simulink model "DTC_Load"  (R2020a)
settings: Solver=VariableStepAuto  StartTime=0.0  StopTime=1  RelTol=1e-3
undefined symbols (not defined in the file): sigbuilder_block
libraries: powerlib x7, simulink x4, mcbcontrolslib x3, mcbpositiondecoderlib x2, powerlib_meascontrol x1
settings Model: Creator=rahee  LastModifiedBy=rahee
settings SolverCC: AlgebraicLoopSolver=LineSearch
settings DataIOCC: ReturnWorkspaceOutputs=off

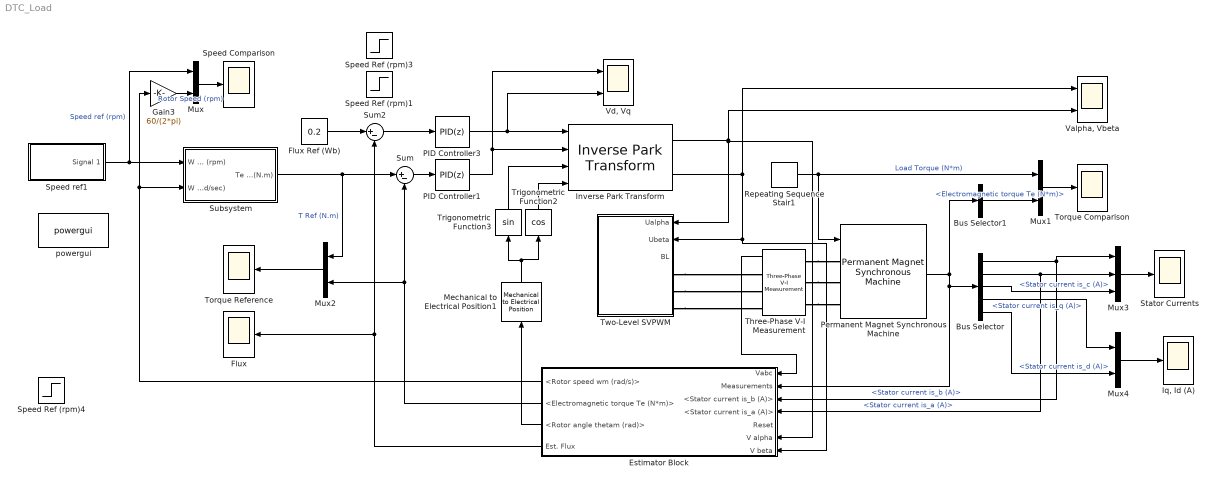
== system DTC_Load ==
  Bus Selector : BusSelector  OutputSignals=Stator current is_b (A),Stator current is_a (A),Stator current is_c (A),Stator current is_q (A),Stator current is_d (A)
  Bus Selector1 : BusSelector  OutputSignals=Electromagnetic torque Te (N*m)
  Estimator Block : Subsystem
  Flux : Scope
  Flux Ref (Wb) : Constant  Value=0.2
  Gain3 : Gain  Gain=60/(2*pi)
  Inverse Park Transform : mcbcontrolslib/Inverse Park Transform  AxisAlignment=D-axis
  "Iq, Id (A)" : Scope
  Mechanical to Electrical Position1 : mcbpositiondecoderlib/Mechanical to Electrical Position  LabelModeActiveChoice=floating-point  NrPP=3  selectedRange=Radians  MechOfstInputType=Specify via dialog  mechOffsetIn=0  maxAngleIn=2*pi  InputDataType=double  VariantSelect=floating-point
      settings: SourceProductBaseCode=MT
  Mux{,1..2,4} (4 alike) : Mux  Inputs=2
  Mux3 : Mux  Inputs=3
  PID Controller1 : simulink/Continuous/PID Controller  Controller=PID  Form=Parallel  TimeDomain=Discrete-time  UseExternalTs=off  SampleTime=-1  IntegratorMethod=Forward Euler  FilterMethod=Forward Euler  ControllerParametersSource=internal  P=8  I=2  D=0  UseFilter=on  N=100  TunerSelectOption=Transfer Function Based (PID Tuner App)  InitialConditionSource=internal  InitialConditionForIntegrator=0  InitialConditionForFilter=0  DifferentiatorICPrevScaledInput=0  ExternalReset=none  TrackingMode=off  Kt=1  LimitOutput=on  UpperSaturationLimit=300  LowerSaturationLimit=-300  LinearizeAsGain=on  AntiWindupMode=clamping  Kb=1  POutMin=[]  POutMax=[]  IOutMin=[]  IOutMax=[]  DOutMin=[]  DOutMax=[]  NOutMin=[]  NOutMax=[]  SumOutMin=[]  SumOutMax=[]  SaturationOutMin=[]  SaturationOutMax=[]  PParamMin=[]  PParamMax=[]  IParamMin=[]  IParamMax=[]  DParamMin=[]  DParamMax=[]  NParamMin=[]  NParamMax=[]  KbParamMin=[]  KbParamMax=[]  KtParamMin=[]  KtParamMax=[]  KbOutMin=[]  KbOutMax=[]  KtOutMin=[]  KtOutMax=[]  IntegratorOutMin=[]  IntegratorOutMax=[]  FilterOutMin=[]  FilterOutMax=[]  SumI1OutMin=[]  SumI1OutMax=[]  SumI2OutMin=[]  SumI2OutMax=[]  SumI3OutMin=[]  SumI3OutMax=[]  SumI4OutMin=[]  SumI4OutMax=[]  SumDOutMin=[]  SumDOutMax=[]  DifferentiatorOutMin=[]  DifferentiatorOutMax=[]  FilterDiffOutCoefMin=[]  FilterDiffOutCoefMax=[]  ReciprocalOutMin=[]  ReciprocalOutMax=[]  SumDenOutMin=[]  SumDenOutMax=[]  SumNumOutMin=[]  SumNumOutMax=[]  DivideOutMin=[]  DivideOutMax=[]  UdiffTsProdOutMin=[]  UdiffTsProdOutMax=[]  NTsProdOutMin=[]  NTsProdOutMax=[]  UintegralTsProdOutMin=[]  UintegralTsProdOutMax=[]  UngainTsProdOutMin=[]  UngainTsProdOutMax=[]  IntegratorContinuousStateAttributes=''  IntegratorStateMustResolveToSignalObject=off  IntegratorRTWStateStorageClass=Auto  FilterContinuousStateAttributes=''  FilterStateMustResolveToSignalObject=off  FilterRTWStateStorageClass=Auto  ParallelPVariant=InternalParameters  IdealPVariant=Disabled  IVariant=InternalParameters  DVariant=InternalParameters  IntegratorVariant=Discrete  SatVariant=Enabled  AWVariant=DiscClampingParallel  PCopyVariant=Disabled  TRVariant=Disabled  FdbkBlocksVariant=Forward  IdealPFdbkVariant=Disabled  SatFdbkVariant=Disabled  DerivativeFilterVariant=ForwardEulerFilter  NVariant=InternalParameters  NCopyVariant=Disabled  FilterICVariant=InternalICsFilter  IntegratorICVariant=InternalICs  ExternalResetVariant=Disabled  TRSumVariant=Passthrough  SumFdbkVariant=Disabled  SumVariant=Sum_PID  TsampFilterVariant=InternalTs  TsampNgainVariant=Passthrough  TsampIntegralVariant=Passthrough
  PID Controller3 : simulink/Continuous/PID Controller  Controller=PID  Form=Parallel  TimeDomain=Discrete-time  UseExternalTs=off  SampleTime=-1  IntegratorMethod=Forward Euler  FilterMethod=Forward Euler  ControllerParametersSource=internal  P=20  I=12  D=0  UseFilter=on  N=100  TunerSelectOption=Transfer Function Based (PID Tuner App)  InitialConditionSource=internal  InitialConditionForIntegrator=0  InitialConditionForFilter=0  DifferentiatorICPrevScaledInput=0  ExternalReset=none  TrackingMode=off  Kt=1  LimitOutput=on  UpperSaturationLimit=300  LowerSaturationLimit=-300  LinearizeAsGain=on  AntiWindupMode=clamping  Kb=1  POutMin=[]  POutMax=[]  IOutMin=[]  IOutMax=[]  DOutMin=[]  DOutMax=[]  NOutMin=[]  NOutMax=[]  SumOutMin=[]  SumOutMax=[]  SaturationOutMin=[]  SaturationOutMax=[]  PParamMin=[]  PParamMax=[]  IParamMin=[]  IParamMax=[]  DParamMin=[]  DParamMax=[]  NParamMin=[]  NParamMax=[]  KbParamMin=[]  KbParamMax=[]  KtParamMin=[]  KtParamMax=[]  KbOutMin=[]  KbOutMax=[]  KtOutMin=[]  KtOutMax=[]  IntegratorOutMin=[]  IntegratorOutMax=[]  FilterOutMin=[]  FilterOutMax=[]  SumI1OutMin=[]  SumI1OutMax=[]  SumI2OutMin=[]  SumI2OutMax=[]  SumI3OutMin=[]  SumI3OutMax=[]  SumI4OutMin=[]  SumI4OutMax=[]  SumDOutMin=[]  SumDOutMax=[]  DifferentiatorOutMin=[]  DifferentiatorOutMax=[]  FilterDiffOutCoefMin=[]  FilterDiffOutCoefMax=[]  ReciprocalOutMin=[]  ReciprocalOutMax=[]  SumDenOutMin=[]  SumDenOutMax=[]  SumNumOutMin=[]  SumNumOutMax=[]  DivideOutMin=[]  DivideOutMax=[]  UdiffTsProdOutMin=[]  UdiffTsProdOutMax=[]  NTsProdOutMin=[]  NTsProdOutMax=[]  UintegralTsProdOutMin=[]  UintegralTsProdOutMax=[]  UngainTsProdOutMin=[]  UngainTsProdOutMax=[]  IntegratorContinuousStateAttributes=''  IntegratorStateMustResolveToSignalObject=off  IntegratorRTWStateStorageClass=Auto  FilterContinuousStateAttributes=''  FilterStateMustResolveToSignalObject=off  FilterRTWStateStorageClass=Auto  ParallelPVariant=InternalParameters  IdealPVariant=Disabled  IVariant=InternalParameters  DVariant=InternalParameters  IntegratorVariant=Discrete  SatVariant=Enabled  AWVariant=DiscClampingParallel  PCopyVariant=Disabled  TRVariant=Disabled  FdbkBlocksVariant=Forward  IdealPFdbkVariant=Disabled  SatFdbkVariant=Disabled  DerivativeFilterVariant=ForwardEulerFilter  NVariant=InternalParameters  NCopyVariant=Disabled  FilterICVariant=InternalICsFilter  IntegratorICVariant=InternalICs  ExternalResetVariant=Disabled  TRSumVariant=Passthrough  SumFdbkVariant=Disabled  SumVariant=Sum_PID  TsampFilterVariant=InternalTs  TsampNgainVariant=Passthrough  TsampIntegralVariant=Passthrough
  Permanent Magnet Synchronous Machine : powerlib/Machines/Permanent Magnet Synchronous Machine  NbPhases=3  FluxDistribution=Sinusoidal  RotorType=Salient-pole  MechanicalLoad=Torque Tm  PresetModel=No  ShowDetailedParameters=on  MeasurementBus=off  Resistance=2  Inductance=8.5e-3  dqInductances=[53.24e-3, 53.24e-3]  La=0.000395  MachineConstant=Torque Constant (N.m / A_peak)  Flux=0.20331  VoltageCst=110.6297  TorqueCst=0.9149  Flat=120  Mechanical=[0.0036 0.0011 3 0]  PolePairs=4  InitialConditions=[0,0, 0,0]  InitialConditions5ph=[0 0 0 0 0 0]  RefAngle=Aligned with phase A axis (original Park)  IterativeDiscreteModel=Trapezoidal non iterative  TsBlock=-1  TsPowergui=0
  Repeating Sequence Stair1 : simulink/Sources/Repeating Sequence Stair  OutValues=[0 0].'  tsamp=0.2  OutMin=[]  OutMax=[]  OutDataTypeStr=double  OutputDataTypeScalingMode=double  OutDataType=fixdt(0,8)  ConRadixGroup=Best Precision: Vector-wise  OutScaling=2^-12
  Speed Comparison : Scope
  Speed Ref (rpm)1 : Step  Time=0.02  After=200  SampleTime=0
  Speed Ref (rpm)3 : Step  Time=0.02  Before=0.2  After=0.2  SampleTime=0
  Speed Ref (rpm)4 : Step  Time=0.1  After=800  SampleTime=0
  Speed ref1 : Subsystem  Tag=STV Subsys  LoadFcn=sigbuilder_block('load',[5.4 30 1141.2 522.6 ]);  StartFcn=sigbuilder_block('start');  StopFcn=sigbuilder_block('stop');  ClipboardFcn=sigbuilder_block('clipboard');  mask(Sigbuilder block){tuvar=[0:10]}
      mask help: Simulink:masks:SigbuilderBlock_MD
      mask init:
      | if ~strcmp(get_param(bdroot(gcbh),'SimulationStatus'),'stopped') tuvar = sigbuilder_block('maskInit'); end
      settings: CopyFcn=sigbuilder_block('copy');  DeleteFcn=sigbuilder_block('delete');  ModelCloseFcn=sigbuilder_block('modelClose');  PreSaveFcn=sigbuilder_block('preSave');  PauseFcn=sigbuilder_block('pause');  ContinueFcn=sigbuilder_block('continue');  NameChangeFcn=sigbuilder_block('namechange');  OpenFcn=sigbuilder_block('open',[5.4 30 1141.2 522.6 ]);  CloseFcn=sigbuilder_block('close');
      mask Display: plot(0, 0, 100, 100,[2, 2, 32, 32, 2], [68, 8, 8, 68, 68],[32, 2], [38, 38], [32, 19, 2],[53, 60, 44], [32, 17, 17, 2],[16, 16, 31, 31]);txt = getActiveGroup(gcbh);text(2, 100, txt,'verticalAlignment', 'top');
  Stator Currents : Scope
  Subsystem : Subsystem
  Sum : Sum  Inputs=|+-
  Sum2 : Sum  Inputs=|+-
  Three-Phase V-I Measurement : powerlib/Measurements/Three-Phase V-I Measurement  VoltageMeasurement=phase-to-ground  SetLabelV=off  LabelV=Vabc  Vpu=off  VpuLL=off  CurrentMeasurement=no  SetLabelI=off  LabelI=Iabc  Ipu=off  Pbase=100e6  Vbase=500e3  OutputType=Complex  PhasorSimulation=off  PSBequivalent=0
  Torque Comparison : Scope
  Torque Reference : Scope
  Trigonometric Function2 : Trigonometry  Operator=cos
  Trigonometric Function3 : Trigonometry
  Two-Level SVPWM : Subsystem
  "Valpha, Vbeta" : Scope  NumInputPorts=2
  "Vd, Vq" : Scope  NumInputPorts=2
  powergui : powerlib/powergui  Priority=1  SimulationMode=Discrete  SampleTime=5e-6  frequency=60  Iterations=50  frequencyindice=0  Pbase=100e6  ErrMax=1e-4  UnitsV=kV  UnitsW=MW  buscounter=0  FunctionMessages=off  echomessages=off  EnableUseOfTLC=off  CurrentSourceSwitches=off  DisableSnubberDevices=off  DisableRonSwitches=off  DisableVfSwitches=off  DisplayEquations=off  AutomaticDiscreteSolvers=off  SolverType=Tustin/Backward Euler (TBE)  Interpol=off  ExternalGateDelay=off  methode=off  Ts=100  x0status=blocks  SPID=on  SwTol=0  HookPort=off  NonlinearTolerance=1e-4  nMaxIteration=100  ContinueOnMaxIteration=off  RestoreLinks=warning  ResistiveCurrentMeasurement=off  Frange=[0:2:500]  Ylog=off  Xlog=on  ShowGrid=off  save=off  variable=ZData  structure=0  ZoomFFT=off  StartTime=0.0  cycles=1  DisplayStyle=1  fundamental=60  FreqAxis=off  MaxFrequency=1000  frequencyindicesteady=1  RmsSteady=1  display=off
  wires:
  Permanent Magnet Synchronous Machine/1 -> Estimator Block/2(Measurements), Bus Selector/1, Bus Selector1/1
  Bus Selector/1 -> Estimator Block/3(<Stator current is_b (A)>), Mux3/1  "<Stator current is_b (A)>"
  Bus Selector/2 -> Mux3/2, Estimator Block/4(<Stator current is_a (A)>)  "<Stator current is_a (A)>"
  Inverse Park Transform/1 -> Estimator Block/6(V alpha), Two-Level SVPWM/1(Ualpha), "Valpha, Vbeta"/2
  Inverse Park Transform/2 -> Estimator Block/7(V beta), Two-Level SVPWM/2(Ubeta), "Valpha, Vbeta"/1
  Sum/1 -> PID Controller1/1
  Sum2/1 -> PID Controller3/1
  Trigonometric Function2/1 -> Inverse Park Transform/4
  Trigonometric Function3/1 -> Inverse Park Transform/3
  Flux Ref (Wb)/1 -> Sum2/1
  PID Controller3/1 -> Inverse Park Transform/1, "Vd, Vq"/2
  PID Controller1/1 -> Inverse Park Transform/2, "Vd, Vq"/1
  Mechanical to Electrical Position1/1 -> Trigonometric Function3/1, Trigonometric Function2/1
  Mux/1 -> Speed Comparison/1
  Mux1/1 -> Torque Comparison/1
  Bus Selector1/1 -> Mux1/2  "<Electromagnetic torque Te (N*m)>"
  Gain3/1 -> Mux/2  "Rotor Speed (rpm)"
  Estimator Block/4(Est. Flux) -> Flux/1, Sum2/2
  Estimator Block/2(<Electromagnetic torque Te (N*m)>) -> Mux2/2, Sum/2
  Estimator Block/1(<Rotor speed wm (rad/s)>) -> Subsystem/2(W meas (rad/sec)), Gain3/1
  Three-Phase V-I Measurement/1 -> Estimator Block/1(Vabc)
  Estimator Block/3(<Rotor angle thetam (rad)>) -> Mechanical to Electrical Position1/1
  Mux2/1 -> Torque Reference/1
  Subsystem/1(Te Ref (N.m)) -> Mux2/1, Sum/1  "T Ref (N.m)"
  Speed ref1/1(Signal 1) -> Mux/1, Subsystem/1(W Ref (rpm))  "Speed ref (rpm)"
  Repeating Sequence Stair1/1 -> Mux1/1, Permanent Magnet Synchronous Machine/1  "Load Torque (N*m)"
  Mux3/1 -> Stator Currents/1
  Bus Selector/3 -> Mux3/3  "<Stator current is_c (A)>"
  Mux4/1 -> "Iq, Id (A)"/1
  Bus Selector/4 -> Mux4/1  "<Stator current is_q (A)>"
  Bus Selector/5 -> Mux4/2  "<Stator current is_d (A)>"
  connections:
  Three-Phase V-I Measurement/LConn1 -- Permanent Magnet Synchronous Machine/LConn1
  Three-Phase V-I Measurement/LConn2 -- Permanent Magnet Synchronous Machine/LConn2
  Three-Phase V-I Measurement/LConn3 -- Permanent Magnet Synchronous Machine/LConn3
  Two-Level SVPWM/LConn1 -- Three-Phase V-I Measurement/RConn1
  Two-Level SVPWM/LConn2 -- Three-Phase V-I Measurement/RConn2
  Two-Level SVPWM/LConn3 -- Three-Phase V-I Measurement/RConn3

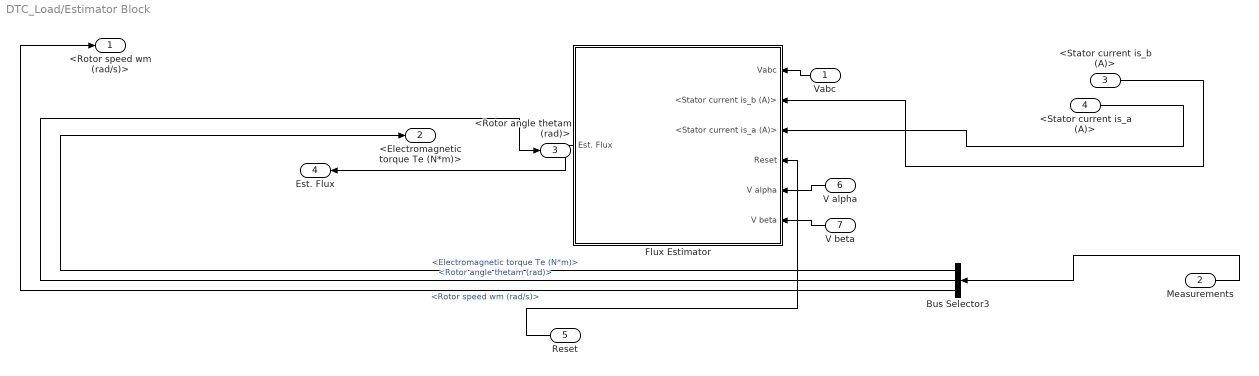
== system DTC_Load/Estimator Block ==
  Vabc : Inport
  Measurements : Inport  Port=2
  <Stator current is_b (A)> : Inport  Port=3
  <Stator current is_a (A)> : Inport  Port=4
  Reset : Inport  Port=5
  V alpha : Inport  Port=6
  V beta : Inport  Port=7
  Bus Selector3 : BusSelector  OutputSignals=Electromagnetic torque Te (N*m),Rotor angle thetam (rad),Rotor speed wm (rad/s)
  Flux Estimator : Subsystem
  <Rotor speed wm (rad/s)> : Outport
  <Electromagnetic torque Te (N*m)> : Outport  Port=2
  <Rotor angle thetam (rad)> : Outport  Port=3
  Est. Flux : Outport  Port=4
  wires:
  Measurements/1 -> Bus Selector3/1
  Bus Selector3/3 -> <Rotor speed wm (rad/s)>/1  "<Rotor speed wm (rad/s)>"
  Flux Estimator/1(Est. Flux) -> Est. Flux/1
  Bus Selector3/1 -> <Electromagnetic torque Te (N*m)>/1  "<Electromagnetic torque Te (N*m)>"
  <Stator current is_a (A)>/1 -> Flux Estimator/3(<Stator current is_a (A)>)
  <Stator current is_b (A)>/1 -> Flux Estimator/2(<Stator current is_b (A)>)
  Vabc/1 -> Flux Estimator/1(Vabc)
  Reset/1 -> Flux Estimator/4(Reset)
  Bus Selector3/2 -> <Rotor angle thetam (rad)>/1  "<Rotor angle thetam (rad)>"
  V alpha/1 -> Flux Estimator/5(V alpha)
  V beta/1 -> Flux Estimator/6(V beta)

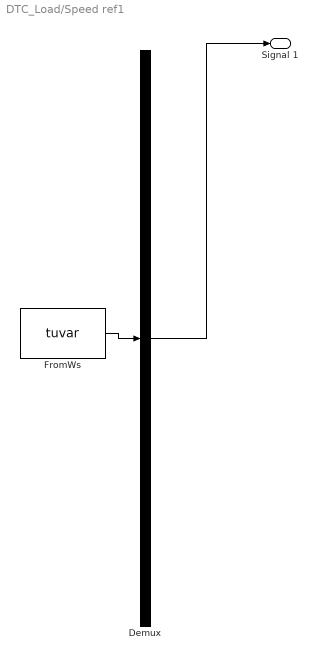
== system DTC_Load/Speed ref1 ==
  Demux : Demux  Tag=STV Demux  Outputs=1
      settings: DisplayOption=none
  FromWs : FromWorkspace  Tag=STV FromWs  VariableName=tuvar  SampleTime=5e-6
      SigBuilderData=|
      | common.afterFinalStr = 'Extrapolate'
      | common.sampleTime = '5e-6'
      | dataSet.timeRange = [0 1]
      | dataSet.name = 'Group 1'
      | sbobj.Groups.Name = 'Group 1'
      | sbobj.Groups.Signals.Name = 'Signal 1'
      | sbobj.Groups.Signals.XData = [0 0.02 0.02 0.6 0.6 1]
      | sbobj.Groups.Signals.YData = [0 0 1800 1800 2000 2000]
      | sbobj.Groups.TimeRange = [0 1]
  Signal 1 : Outport  Tag=STV Outport
  wires:
  FromWs/1 -> Demux/1
  Demux/1 -> Signal 1/1

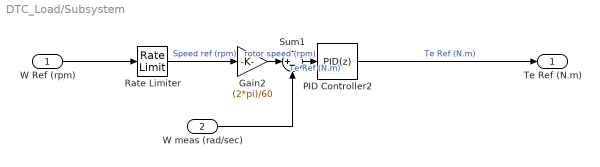
== system DTC_Load/Subsystem ==
  W Ref (rpm) : Inport
  W meas (rad/sec) : Inport  Port=2
  Gain2 : Gain  Gain=(2*pi)/60
  PID Controller2 : simulink/Continuous/PID Controller  Controller=PID  Form=Parallel  TimeDomain=Discrete-time  UseExternalTs=off  SampleTime=-1  IntegratorMethod=Forward Euler  FilterMethod=Forward Euler  ControllerParametersSource=internal  P=8  I=0.8  D=0  UseFilter=on  N=100  TunerSelectOption=Transfer Function Based (PID Tuner App)  InitialConditionSource=internal  InitialConditionForIntegrator=0  InitialConditionForFilter=0  DifferentiatorICPrevScaledInput=0  ExternalReset=none  TrackingMode=off  Kt=1  LimitOutput=on  UpperSaturationLimit=20  LowerSaturationLimit=-20  LinearizeAsGain=on  AntiWindupMode=clamping  Kb=1  POutMin=[]  POutMax=[]  IOutMin=[]  IOutMax=[]  DOutMin=[]  DOutMax=[]  NOutMin=[]  NOutMax=[]  SumOutMin=[]  SumOutMax=[]  SaturationOutMin=[]  SaturationOutMax=[]  PParamMin=[]  PParamMax=[]  IParamMin=[]  IParamMax=[]  DParamMin=[]  DParamMax=[]  NParamMin=[]  NParamMax=[]  KbParamMin=[]  KbParamMax=[]  KtParamMin=[]  KtParamMax=[]  KbOutMin=[]  KbOutMax=[]  KtOutMin=[]  KtOutMax=[]  IntegratorOutMin=[]  IntegratorOutMax=[]  FilterOutMin=[]  FilterOutMax=[]  SumI1OutMin=[]  SumI1OutMax=[]  SumI2OutMin=[]  SumI2OutMax=[]  SumI3OutMin=[]  SumI3OutMax=[]  SumI4OutMin=[]  SumI4OutMax=[]  SumDOutMin=[]  SumDOutMax=[]  DifferentiatorOutMin=[]  DifferentiatorOutMax=[]  FilterDiffOutCoefMin=[]  FilterDiffOutCoefMax=[]  ReciprocalOutMin=[]  ReciprocalOutMax=[]  SumDenOutMin=[]  SumDenOutMax=[]  SumNumOutMin=[]  SumNumOutMax=[]  DivideOutMin=[]  DivideOutMax=[]  UdiffTsProdOutMin=[]  UdiffTsProdOutMax=[]  NTsProdOutMin=[]  NTsProdOutMax=[]  UintegralTsProdOutMin=[]  UintegralTsProdOutMax=[]  UngainTsProdOutMin=[]  UngainTsProdOutMax=[]  IntegratorContinuousStateAttributes=''  IntegratorStateMustResolveToSignalObject=off  IntegratorRTWStateStorageClass=Auto  FilterContinuousStateAttributes=''  FilterStateMustResolveToSignalObject=off  FilterRTWStateStorageClass=Auto  ParallelPVariant=InternalParameters  IdealPVariant=Disabled  IVariant=InternalParameters  DVariant=InternalParameters  IntegratorVariant=Discrete  SatVariant=Enabled  AWVariant=DiscClampingParallel  PCopyVariant=Disabled  TRVariant=Disabled  FdbkBlocksVariant=Forward  IdealPFdbkVariant=Disabled  SatFdbkVariant=Disabled  DerivativeFilterVariant=ForwardEulerFilter  NVariant=InternalParameters  NCopyVariant=Disabled  FilterICVariant=InternalICsFilter  IntegratorICVariant=InternalICs  ExternalResetVariant=Disabled  TRSumVariant=Passthrough  SumFdbkVariant=Disabled  SumVariant=Sum_PID  TsampFilterVariant=InternalTs  TsampNgainVariant=Passthrough  TsampIntegralVariant=Passthrough
  Rate Limiter : RateLimiter  RisingSlewLimit=(2000-0)/(0.088-0)  FallingSlewLimit=-(2000-0)/(0.088-0)  SampleTimeMode=inherited
  Sum1 : Sum  Inputs=|+-
  Te Ref (N.m) : Outport
  wires:
  Gain2/1 -> Sum1/1  "rotor speed (rpm)"
  Sum1/1 -> PID Controller2/1  "Te Ref (N.m)"
  W meas (rad/sec)/1 -> Sum1/2
  PID Controller2/1 -> Te Ref (N.m)/1  "Te Ref (N.m)"
  W Ref (rpm)/1 -> Rate Limiter/1
  Rate Limiter/1 -> Gain2/1  "Speed ref (rpm)"

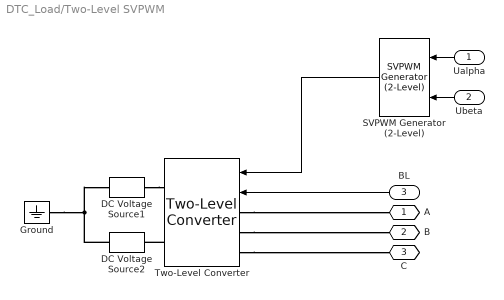
== system DTC_Load/Two-Level SVPWM ==
  Ualpha : Inport
  Ubeta : Inport  Port=2
  BL : Inport  Port=3
  DC Voltage Source1 : powerlib/Electrical Sources/DC Voltage Source  Amplitude=300  Measurements=None
  DC Voltage Source2 : powerlib/Electrical Sources/DC Voltage Source  Amplitude=300  Measurements=None
  Ground : powerlib/Elements/Ground  LConnTagsString=a
  SVPWM Generator (2-Level) : powerlib_meascontrol/Pulse & Signal Generators/SVPWM Generator (2-Level)  InputType=alpha-beta components  SwitchingPattern=Pattern #1  Fc=2000  ParUref=[0.8 -30 50]  Ts=0
      settings: SourceProductBaseCode=PS
  Two-Level Converter : powerlib/Power Electronics/Two-Level Converter  ModelType=Switching devices  Ron=1e-3  Rs=1e6  Cs=inf  Vforward=[0,0]  Ron_Diode=1e-3  Rs_Diode=1e6  Cs_Diode=inf  Vf_Diode=1e-3  Rs_CurrentSource=inf
      settings: SourceProductBaseCode=PS
  A : PMIOPort  Side=Left
  B : PMIOPort  Port=2  Side=Left
  C : PMIOPort  Port=3  Side=Left
  wires:
  SVPWM Generator (2-Level)/1 -> Two-Level Converter/1
  Ubeta/1 -> SVPWM Generator (2-Level)/2
  Ualpha/1 -> SVPWM Generator (2-Level)/1
  BL/1 -> Two-Level Converter/2
  connections:
  Two-Level Converter/RConn2 -- DC Voltage Source2/LConn1
  DC Voltage Source2/RConn1 -- Ground/LConn1 -- DC Voltage Source1/LConn1
  Two-Level Converter/LConn3 -- C/RConn1
  Two-Level Converter/LConn1 -- A/RConn1
  DC Voltage Source1/RConn1 -- Two-Level Converter/RConn1
  Two-Level Converter/LConn2 -- B/RConn1

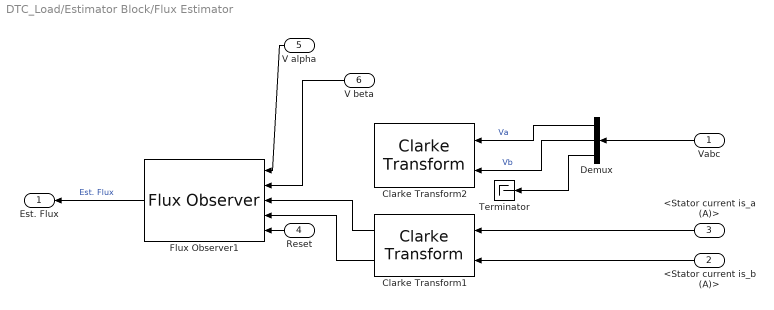
== system DTC_Load/Estimator Block/Flux Estimator ==
  Vabc : Inport
  <Stator current is_b (A)> : Inport  Port=2
  <Stator current is_a (A)> : Inport  Port=3
  Reset : Inport  Port=4
  V alpha : Inport  Port=5
  V beta : Inport  Port=6
  Clarke Transform1 : mcbcontrolslib/Clarke Transform  VariantControl=Variant2
  Clarke Transform2 : mcbcontrolslib/Clarke Transform  VariantControl=Variant2
  Demux : Demux  Outputs=3
  Flux Observer1 : mcbpositiondecoderlib/Flux Observer  BlockInputUnit=SI unit  PerUnitVoltage=13.86  PerUnitCurrent=19.3  PositionSelect=off  FluxSelect=on  TorqueSelect=off  PolePairs=3  StatorResistance=2  BlockSampleTime=5e-6  PositionUnit=Radians  PositionDatatype=double  FluxUnit=Weber  PerUnitFlux=0.1  FluxDatatype=double  TorqueUnit=Nm  PerUnitTorque=100  TorqueDatatype=double
      settings: SourceProductBaseCode=MT
  Terminator : Terminator
  Est. Flux : Outport
  wires:
  Vabc/1 -> Demux/1
  Demux/3 -> Terminator/1
  Clarke Transform1/1 -> Flux Observer1/3
  Clarke Transform1/2 -> Flux Observer1/4
  Demux/1 -> Clarke Transform2/1  "Va"
  Flux Observer1/1 -> Est. Flux/1  "Est. Flux"
  Demux/2 -> Clarke Transform2/2  "Vb"
  <Stator current is_b (A)>/1 -> Clarke Transform1/2
  <Stator current is_a (A)>/1 -> Clarke Transform1/1
  Reset/1 -> Flux Observer1/5
  V beta/1 -> Flux Observer1/2
  V alpha/1 -> Flux Observer1/1
